simulink model "sldemo_tc_blocks"  (R2024a)
settings: Solver=FixedStepDiscrete  StartTime=0.0  StopTime=1  FixedStep=1  RelTol=1e-3  EnableMultiTasking=on
model workspace: external: MAT-File sldemo_tc_blocks_data.mat (data not in the file)
undefined symbols (not defined in the file): TypeB_degC, TypeB_Volts, TypeE_degC, TypeE_Volts, TypeJ_degC, TypeJ_Volts, TypeK_degC, TypeK_Volts, TypeN_degC, TypeN_Volts, TypeR_degC, TypeR_Volts, TypeT_degC, TypeT_Volts
Description:
  | ITS-90 Thermocouple Models
  | 
  | Full-Range 2 degrees Celsius Interpolated Thermocouple Tables created using
  | one ITS-90 Interpolating Polynomial and one inverse polynomial per junction type.
settings Model: Creator=The MathWorks, Inc.  LastModifiedBy=neham
settings SolverCC: AlgebraicLoopSolver=TrustRegion
settings DataIOCC: LimitDataPoints=on  SaveFormat=Array
settings OptimizationCC: BlockReduction=off  ConditionallyExecuteInputs=off  OptimizeBlockIOStorage=off  BufferReuse=off  GlobalBufferReuse=off  ExpressionFolding=off  ExpressionDepthLimit=2147483647  LocalBlockOutputs=off  InitFltsAndDblsToZero=on  EfficientMapNaN2IntZero=off  LifeSpan=inf  BufferReusableBoundary=off  OptimizeDataStoreBuffers=off  BusAssignmentInplaceUpdate=off
settings DebuggingCC: UnderspecifiedInitializationDetection=Classic  MergeDetectMultiDrivingBlocksExec=none  CheckExecutionContextPreStartOutputMsg=on  SignalResolutionControl=TryResolveAllWithWarning  MultiTaskDSMMsg=warning  MultiTaskCondExecSysMsg=none  FcnCallInpInsideContextMsg=warning  UnconnectedLineMsg=warning  BusObjectLabelMismatch=none  StateNameClashWarn=warning  SFUnexpectedBacktrackingDiag=warning  SFNoUnconditionalDefaultTransitionDiag=warning  SFExecutionAtInitializationDiag=none  ArithmeticOperatorsInVariantConditions=warning
settings HardwareCC: ProdBitPerPointer=32  ProdBitPerSizeT=32  ProdBitPerPtrDiffT=32  ProdLargestAtomicFloat=None  ProdIntDivRoundTo=Undefined  ProdEndianess=Unspecified  ProdWordSize=32  ProdHWDeviceType=32-bit Generic
settings ModelReferenceCC: EnableRefExpFcnMdlSchedulingChecks=on  PropagateSignalLabelsOutOfModel=off
settings SFSimCC: SimUseLocalCustomCode=off  CustomCodeUndefinedFunction=UseInterfaceOnly
settings RTWCC: RTWUseLocalCustomCode=off  GPUComputeCapability=3.5
settings CodeAppCC: StateflowObjectComments=on
settings GRTTargetCC: TargetFcnLib=ansi_tfl_tmw_new.mat  TargetLangStandard=C89/C90 (ANSI)  CombineOutputUpdateFcns=off  GRTInterface=on
settings ConfigComp: CovMetricSettings=dw  CovSaveCumulativeToWorkspaceVar=on  CovSaveSingleToWorkspaceVar=on  CovExternalEMLEnable=off

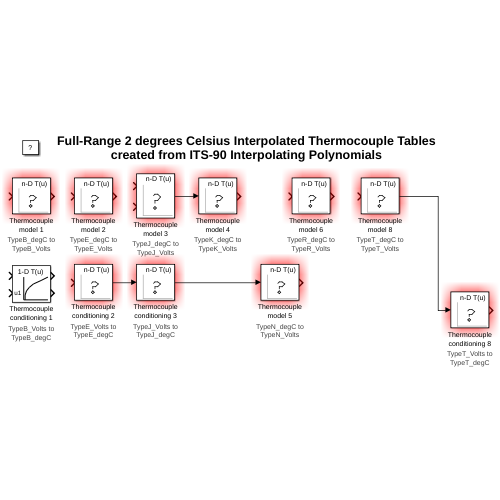
[thumbnail: Simulink's stored preview of the top-level diagram]
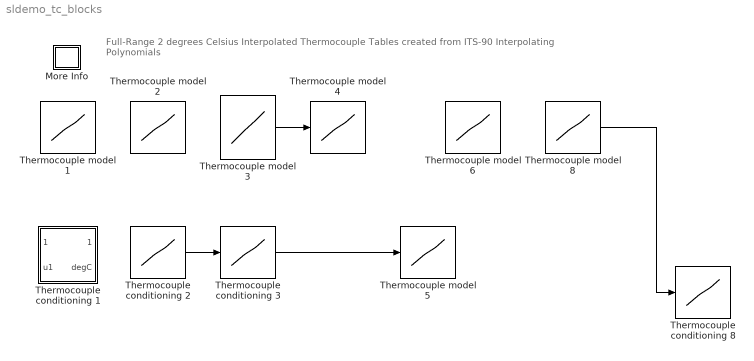
== system sldemo_tc_blocks ==
  note: Full-Range 2 degrees Celsius Interpolated Thermocouple Tables
      | created from ITS-90 Interpolating Polynomials
  More Info : Subsystem
      settings: OpenFcn=showExample('simulink_general/sldemo_tc_scriptExample')
      mask Display: disp('?')
  Thermocouple conditioning 1 : Subsystem
      settings: AttributesFormatString=TypeB_Volts to\nTypeB_degC
      mask Display:
      | text(.15,.85,'1-D T(u)')
      | plot([0.3 0.3 0.95],[0.7 0.05 0.05])
      | plot([0.95 0.7515 0.554 0.4535 0.375 0.335 0.325],[0.7 0.6 0.5 0.4 0.3 0.2 0.05])
  Thermocouple conditioning 2 : Lookup_n-D  NumberOfTableDimensions=1  BreakpointsForDimension1=TypeE_Volts  BeginIndexSearchUsingPreviousIndexResult=on  Table=TypeE_degC  DiagnosticForOutOfRangeInput=Warning
      settings: AttributesFormatString=%<bp1> to\n%<tableData>
  Thermocouple conditioning 3 : Lookup_n-D  NumberOfTableDimensions=1  BreakpointsForDimension1=TypeJ_Volts  BeginIndexSearchUsingPreviousIndexResult=on  Table=TypeJ_degC  DiagnosticForOutOfRangeInput=Warning
      settings: AttributesFormatString=%<bp1> to\n%<tableData>
  Thermocouple conditioning 8 : Lookup_n-D  NumberOfTableDimensions=1  BreakpointsForDimension1=TypeT_Volts  BeginIndexSearchUsingPreviousIndexResult=on  Table=TypeT_degC  DiagnosticForOutOfRangeInput=Warning
      settings: AttributesFormatString=%<bp1> to\n%<tableData>
  Thermocouple model 1 : Lookup_n-D  NumberOfTableDimensions=1  BreakpointsForDimension1=TypeB_degC  BeginIndexSearchUsingPreviousIndexResult=on  Table=TypeB_Volts  DiagnosticForOutOfRangeInput=Warning
      settings: AttributesFormatString=%<bp1> to\n%<tableData>
  Thermocouple model 2 : Lookup_n-D  NumberOfTableDimensions=1  BreakpointsForDimension1=TypeE_degC  BeginIndexSearchUsingPreviousIndexResult=on  Table=TypeE_Volts  DiagnosticForOutOfRangeInput=Warning
      settings: AttributesFormatString=%<bp1> to\n%<tableData>
  Thermocouple model 3 : Lookup_n-D  BreakpointsForDimension1=TypeJ_degC  BeginIndexSearchUsingPreviousIndexResult=on  Table=TypeJ_Volts  DiagnosticForOutOfRangeInput=Warning
      settings: AttributesFormatString=%<bp1> to\n%<tableData>  InputPortMap=u0,u1
  Thermocouple model 4 : Lookup_n-D  NumberOfTableDimensions=1  BreakpointsForDimension1=TypeK_degC  BeginIndexSearchUsingPreviousIndexResult=on  Table=TypeK_Volts  DiagnosticForOutOfRangeInput=Warning
      settings: AttributesFormatString=%<bp1> to\n%<tableData>
  Thermocouple model 5 : Lookup_n-D  NumberOfTableDimensions=1  BreakpointsForDimension1=TypeN_degC  BeginIndexSearchUsingPreviousIndexResult=on  Table=TypeN_Volts  DiagnosticForOutOfRangeInput=Warning
      settings: AttributesFormatString=%<bp1> to\n%<tableData>
  Thermocouple model 6 : Lookup_n-D  NumberOfTableDimensions=1  BreakpointsForDimension1=TypeR_degC  BeginIndexSearchUsingPreviousIndexResult=on  Table=TypeR_Volts  DiagnosticForOutOfRangeInput=Warning
      settings: AttributesFormatString=%<bp1> to\n%<tableData>
  Thermocouple model 8 : Lookup_n-D  NumberOfTableDimensions=1  BreakpointsForDimension1=TypeT_degC  BeginIndexSearchUsingPreviousIndexResult=on  Table=TypeT_Volts  DiagnosticForOutOfRangeInput=Warning
      settings: AttributesFormatString=%<bp1> to\n%<tableData>
  wires:
  Thermocouple conditioning 2/1 -> Thermocouple conditioning 3/1
  Thermocouple model 3/1 -> Thermocouple model 4/1
  Thermocouple model 8/1 -> Thermocouple conditioning 8/1
  Thermocouple conditioning 3/1 -> Thermocouple model 5/1

== system sldemo_tc_blocks/More Info ==

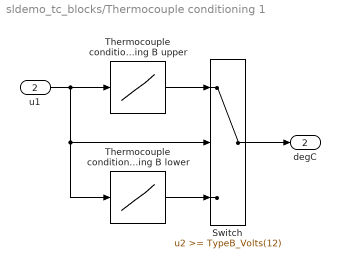
== system sldemo_tc_blocks/Thermocouple conditioning 1 ==
  u1 : Inport  Port=2
  Switch : Switch  Threshold=TypeB_Volts(12)  SaturateOnIntegerOverflow=off  InputSameDT=off
  Thermocouple conditioning B lower : Lookup_n-D  NumberOfTableDimensions=1  BreakpointsForDimension1=TypeB_Volts(12:-1:1)  BeginIndexSearchUsingPreviousIndexResult=on  Table=TypeB_degC(12:-1:1)  DiagnosticForOutOfRangeInput=Warning
      settings: AttributesFormatString=%<bp1> to\n%<tableData>
  Thermocouple conditioning B upper : Lookup_n-D  NumberOfTableDimensions=1  BreakpointsForDimension1=TypeB_Volts(12:end)  BeginIndexSearchUsingPreviousIndexResult=on  Table=TypeB_degC(12:end)  DiagnosticForOutOfRangeInput=Warning
      settings: AttributesFormatString=%<bp1> to\n%<tableData>
  degC : Outport  Port=2  VectorParamsAs1DForOutWhenUnconnected=off
  wires:
  Switch/1 -> degC/1
  Thermocouple conditioning B lower/1 -> Switch/3
  Thermocouple conditioning B upper/1 -> Switch/1
  u1/1 -> Switch/2, Thermocouple conditioning B lower/1, Thermocouple conditioning B upper/1
